simulink model "FindLeadCar"  (R2024a)
settings: configuration reference "csMultiInstance" (kept outside this file)
undefined symbols (not defined in the file or in its folder): LaneWidth, posSelector, Ts
Description:
  | Model to find leading car from information about other traffic participants and lane boundaries. This is considered as a SW unit.
settings Model: DataDictionary=DD_FindLeadCar.sldd  EnableAccessToBaseWorkspace=off  Creator=The MathWorks, Inc.  LastModifiedBy=The MathWorks, Inc.
settings ConfigSetRef: SourceName=csMultiInstance

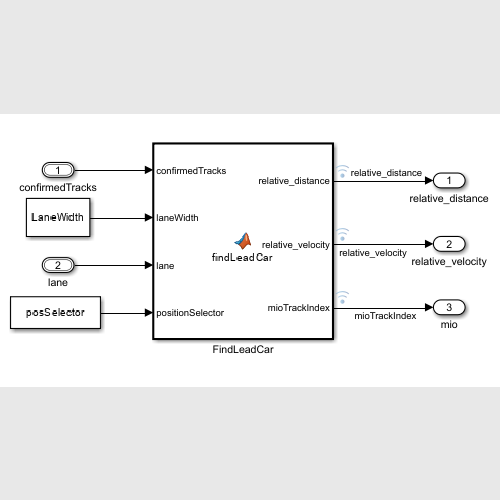
[thumbnail: Simulink's stored preview of the top-level diagram]
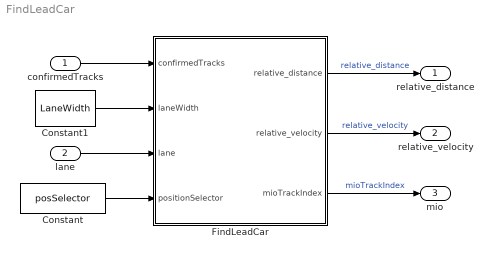
== system FindLeadCar ==
  confirmedTracks : Inport  OutDataTypeStr=Bus: BusMultiObjectTracker  PortDimensions=[1 1]  SampleTime=Ts  BusOutputAsStruct=on
  lane : Inport  Port=2  OutDataTypeStr=Bus: LaneSensor  PortDimensions=[1 1]  SampleTime=Ts  BusOutputAsStruct=on
  Constant : Constant  Value=posSelector
  Constant1 : Constant  Value=LaneWidth
  FindLeadCar : MATLAB Function  TreatAsAtomicUnit=on
  relative_distance : Outport  OutDataTypeStr=double  PortDimensions=1  SampleTime=Ts
  relative_velocity : Outport  Port=2  OutDataTypeStr=double  PortDimensions=1  SampleTime=Ts
  mio : Outport  Port=3  OutDataTypeStr=double  PortDimensions=1  SampleTime=Ts
  wires:
  FindLeadCar/2(relative_velocity) -> relative_velocity/1  "relative_velocity"
  FindLeadCar/3(mioTrackIndex) -> mio/1  "mioTrackIndex"
  lane/1 -> FindLeadCar/3(lane)
  FindLeadCar/1(relative_distance) -> relative_distance/1  "relative_distance"
  confirmedTracks/1 -> FindLeadCar/1(confirmedTracks)
  Constant/1 -> FindLeadCar/4(positionSelector)
  Constant1/1 -> FindLeadCar/2(laneWidth)

== matlab function FindLeadCar/FindLeadCar ==
  data: confirmedTracks input; laneWidth input; relative_distance output size=[1 1]; relative_velocity output size=[1 1]; lane input; mioTrackIndex output; positionSelector input
    function [relative_distance,relative_velocity,mioTrackIndex] = findLeadCar(confirmedTracks, laneWidth, lane, positionSelector)
% This function finds the lead car: a car in front of the ego car that
% satisfies all the criteria below:
% * Within the ego car's lane.
% * In front of the ego car.
% * Closest to the ego car.

% Note: If you change state definition, change the following:
%       State = [x;vx;y;vy;z;vz] (3D constant velocity)
numStates = 6;
numTracks = confirmedTracks.NumTracks;
% Initialize outputs and parameters
egoVehicleIdx = uint8(1);
maxX = cast(1000, 'like', confirmedTracks.Tracks(egoVehicleIdx).State);  % Far enough forward so that no track is expected to exceed this distance
mioTrackIndex = 0;

% If lane detection is not available, the ego car is assumed to be located
% in the middle of its lane. The lane width is assumed to be 3.6m, typical
% highway lane width.
    
halfLaneWidth = laneWidth/2;

if lane.Left.Strength > 0.01
    lb = [lane.Left.CurvatureDerivative/6,...
        lane.Left.Curvature/2,...
        lane.Left.HeadingAngle,...
        lane.Left.LateralOffset];
else
    lb = single([0,0,0,halfLaneWidth]);
end

if lane.Right.Strength > 0.01
    rb = [lane.Right.CurvatureDerivative/6,...
        lane.Right.Curvature/2,...
        lane.Right.HeadingAngle,...
        lane.Right.LateralOffset];
else
    rb = single([0,0,0,-halfLaneWidth]);    
end

for i = 1:numTracks
    position = positionSelector * confirmedTracks.Tracks(i).State;
    relative_distance = position(uint8(1)); % Longitudinal position of the track relative to ego
    y = single(position(uint8(2))); % Lateral position of the track relative to ego
    
    if relative_distance < maxX && relative_distance > 0 % No point checking otherwise

        yleftLane  = polyval(lb,relative_distance); % lateral position of left lane
        yrightLane = polyval(rb,relative_distance); % lateral position of right lane
        
        % Find a new lead car
        if (yrightLane <= y) && (y <= yleftLane)
            maxX = relative_distance;
            mioTrackIndex = i;
        end
    end
end

if mioTrackIndex>0
    mioState = confirmedTracks.Tracks(mioTrackIndex).State;
else
    mioState = 10000*ones(numStates,1,'like',confirmedTracks.Tracks(egoVehicleIdx).State);
end

% Output:
relative_distance = mioState(uint8(1));    % Longitudinal position of the lead car
relative_velocity = mioState(uint8(2));   % Longitudinal velocity of the lead car
